simulink model "simulateDBPSK"  (R2023b)
settings: Solver=VariableStepAuto  StartTime=0.0  StopTime=5  RelTol=1e-3
libraries: commdigbbndpm3 x2, commchan3 x1, commrandsrc3 x1, commsink2 x1, commrflib2 x1, dspsrcs4 x1
settings Model: Creator=prust  LastModifiedBy=龚玲玉
settings SolverCC: AlgebraicLoopSolver=TrustRegion
settings DataIOCC: ReturnWorkspaceOutputs=off
settings DebuggingCC: UnconnectedInputMsg=warning  UnconnectedOutputMsg=warning  UnconnectedLineMsg=warning  ArithmeticOperatorsInVariantConditions=warning
settings ModelReferenceCC: EnableRefExpFcnMdlSchedulingChecks=on
settings SFSimCC: SimUseLocalCustomCode=off  CustomCodeUndefinedFunction=UseInterfaceOnly
settings RTWCC: RTWUseLocalCustomCode=off  DLArmComputeVersion=19.05
settings CodeAppCC: StateflowObjectComments=on

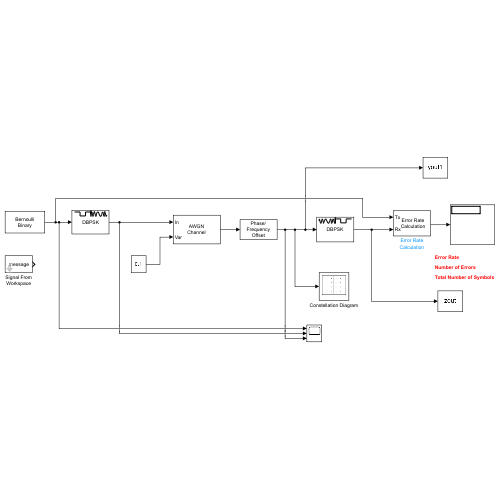
[thumbnail: Simulink's stored preview of the top-level diagram]
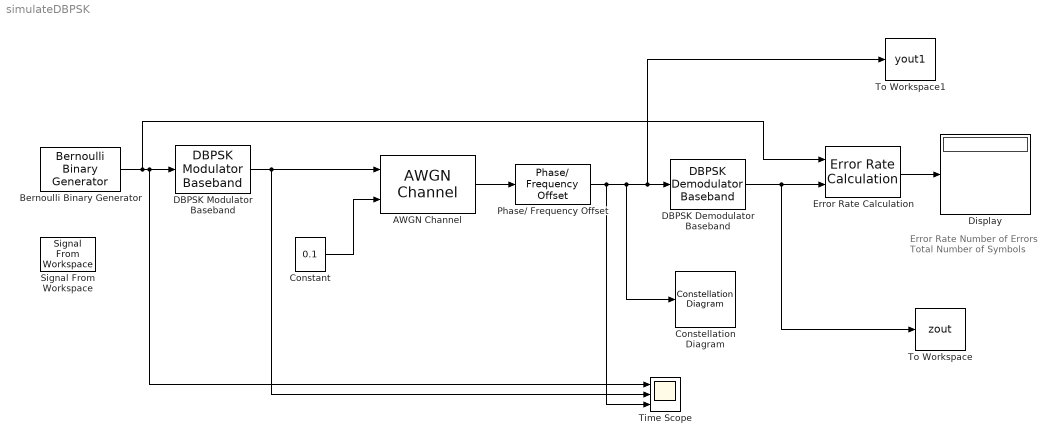
== system simulateDBPSK ==
  note: Error Rate
      |
      | Number of Errors
      |
      | Total Number of Symbols
  AWGN Channel : commchan3/AWGN Channel  LegacyMode=on  NoiseMethod="Signal to noise ratio  (SNR)"  noiseMode=Variance from port  EbNo=50  EsNo=10  SNR=10  BitsPerSymbol=1  SignalPower=1  SamplesPerSymbol=1  SymbolPeriod=1/8000  VarianceSource=Parameter  Variance=1  RandomStream=Global stream  Seed=67  SimulateUsing=Code generation
  Bernoulli Binary Generator : commrandsrc3/Bernoulli Binary Generator  ProbabilityOfZero=0.5  SeedSource=Auto  Seed=0  SampleTime=1/8000  SamplesPerFrame=1000  OutputDataType=double  SimulateUsing=Interpreted execution
  Constant : Constant  Value=0.1  VectorParams1D=off
  Constellation Diagram : ConstellationDiagram  WindowPosition=[1082.000000,91.000000,341.000000,345.000000,]  ScopeFrameLocation=window  ReferenceConstellation=BPSK  XLimits=[-2.6078 2.6529]  YLimits=[-2.6078 2.6529]  DefaultConfigurationName=comm.scopes.ConstellationDiagramBlockCfg
  DBPSK Demodulator Baseband : commdigbbndpm3/DBPSK Demodulator Baseband  Ph=0  outDtype=Inherit via internal rule
  DBPSK Modulator Baseband : commdigbbndpm3/DBPSK Modulator Baseband  Ph=0  outDtype=double
  Display : Display
  Error Rate Calculation : commsink2/Error Rate Calculation  N=0  st_delay=0  cp_mode=Entire frame  subframe=[]  PMode=Port  WsName=ErrorVec  RsMode2=off  stop=off  numErr=100  maxBits=1e6
  Phase/ Frequency Offset : commrflib2/Phase// Frequency Offset  phaseOffset=0  freqPort=off  freqOffset=0
  Signal From Workspace : dspsrcs4/Signal From Workspace  X=message  Ts=1/8e3  nsamps=30000  OutputAfterFinalValue=Cyclic repetition  ignoreOrWarnInputAndFrameLengths=off  OutputFrames=off
  Time Scope : Scope  NumInputPorts=3
  To Workspace : ToWorkspace  VariableName=zout  SampleTime=-1
      settings: MaxDataPoints=2560  Save2DSignal=2-D array (concatenate along first dimension)
  To Workspace1 : ToWorkspace  VariableName=yout1  SampleTime=-1
      settings: MaxDataPoints=2560  Save2DSignal=2-D array (concatenate along first dimension)
  wires:
  DBPSK Modulator Baseband/1 -> AWGN Channel/1, Time Scope/2
  AWGN Channel/1 -> Phase/ Frequency Offset/1
  DBPSK Demodulator Baseband/1 -> To Workspace/1, Error Rate Calculation/2
  Error Rate Calculation/1 -> Display/1
  Phase/ Frequency Offset/1 -> Time Scope/3, Constellation Diagram/1, To Workspace1/1, DBPSK Demodulator Baseband/1
  Constant/1 -> AWGN Channel/2
  Bernoulli Binary Generator/1 -> Error Rate Calculation/1, Time Scope/1, DBPSK Modulator Baseband/1
